simulink model "testemplanner_cs"  (R2023a)
settings: Solver=ode5  StartTime=0.0  StopTime=60  FixedStep=1/1000  RelTol=1e-3
PreLoadFcn:
  | mbxruntime.callbacks.PreLoadFcn(bdroot);
PostLoadFcn:
  | mbxruntime.callbacks.PostLoadFcn(bdroot);
InitFcn:
  | mbxruntime.callbacks.InitFcn(bdroot);
StartFcn:
  | mbxruntime.callbacks.StartFcn(bdroot);
StopFcn:
  | mbxruntime.callbacks.StopFcn(bdroot);
model workspace (MAT data in the model file):
  mbox_table : object (value not decoded)
  model_closed = 0
  sim_status = 0
undefined symbols (not defined in the file): aubr, c_factor, cf, cr, DiscIntNeverNeededParam, global_path_x, global_path_y, KD_PID_distance, KD_PID_speed, KI_PID_distance, KI_PID_speed, KP_PID_distance, KP_PID_speed, la, lb, LQR_K1, LQR_K2, LQR_K3, LQR_K4, m, rack_displacement, right_wheel_ground, tablebr, vubr, vx_break_point
libraries: PreScanSimulinkLibrary x14, Solver_SF x1
(part 8 of 8)

== matlab function testemplanner_cs/Audi_A8_Sedan_1/decision&planning module1/referenceline provider/MATLAB Function ==
  data: path_x input; path_heading output; path_y input; path_kappa output
function [path_heading, path_kappa] = fcn(path_x, path_y)

%原理：heading=atan(dy/dx)
%kappa=dheading/ds
%ds=(dx^2+dy^2)^0.5
%但角度存在多值性问题，例如heading=atan(dy/dx)=heading+pi,在三角函数运算时会出现问题
%可以容忍heading+2pi（三角函数运算不会出现问题），但计算kappa=(dheading+2pi)/ds时要做特殊处理
%很多奇怪问题的根源就是角度的多值性处理不当
%中点欧拉法不能直接用

%dx,dy而不是角度用中点欧拉
dx = diff(path_x);
dy = diff(path_y);

dx_pre = [dx(1);dx];
dx_end = [dx;dx(end)];
dx_final = (dx_pre+dx_end)/2;

dy_pre = [dy(1);dy];
dy_end = [dy;dy(end)];
dy_final = (dy_pre+dy_end)/2;

%.^2是对每一个元素做平方运算，^2是矩阵运算
ds_final = sqrt(dx_final.^2+dy_final.^2);

%atan2为四象限反正切，将角度限定在-pi-pi
path_heading = atan2(dy_final,dx_final);

%对heading做差分，得到dheading，同样采用中点欧拉
dheading = diff(path_heading);
dheading_pre = [dheading(1);dheading];
dheading_after = [dheading;dheading(end)];
dheading_final = (dheading_pre+dheading_after)/2;

%认为dheading为很小量，用sin(dheading)近似代替heading,因为sin(dheading)与sin(dheading+2pi)相等
path_kappa = dheading_final./ds_final;

== matlab function testemplanner_cs/Audi_A8_Sedan_1/decision&planning module1/referenceline provider/MATLAB Function1 ==
  data: host_match_point_index input; referenceline_x_init output; global_path_x input; global_path_y input; referenceline_y_init output
function [referenceline_x_init, referenceline_y_init] = fcn(host_match_point_index, global_path_x, global_path_y)

%提取未经过优化的全局路径
%从自车的匹配点开始，向前取150个点，向后取30个点，总共181个点
%如果后面的点不够30...
%如果前面的点不够150...
%满足条件

start_index = -1;
%后面不足30个点
if host_match_point_index-30 < 1
    start_index = 1;
elseif host_match_point_index+180 > length(global_path_x)
    start_index = length(global_path_x)-180;
else
    start_index = host_match_point_index-29;%可能有问题
end

referenceline_x_init = global_path_x(start_index:start_index+180);
referenceline_y_init = global_path_y(start_index:start_index+180);

== matlab function testemplanner_cs/Audi_A8_Sedan_1/decision&planning module1/referenceline provider/MATLAB Function2 ==
  data: path_x input; path_heading output; path_y input; path_kappa output
function [path_heading, path_kappa] = fcn(path_x, path_y)

%原理：heading=atan(dy/dx)
%kappa=dheading/ds
%ds=(dx^2+dy^2)^0.5
%但角度存在多值性问题，例如heading=atan(dy/dx)=heading+pi,在三角函数运算时会出现问题
%可以容忍heading+2pi（三角函数运算不会出现问题），但计算kappa=(dheading+2pi)/ds时要做特殊处理
%很多奇怪问题的根源就是角度的多值性处理不当
%中点欧拉法不能直接用

%dx,dy而不是角度用中点欧拉
dx = diff(path_x);
dy = diff(path_y);

dx_pre = [dx(1);dx];
dx_end = [dx;dx(end)];
dx_final = (dx_pre+dx_end)/2;

dy_pre = [dy(1);dy];
dy_end = [dy;dy(end)];
dy_final = (dy_pre+dy_end)/2;

%.^2是对每一个元素做平方运算，^2是矩阵运算
ds_final = sqrt(dx_final.^2+dy_final.^2);

%atan2为四象限反正切，将角度限定在-pi-pi
path_heading = atan2(dy_final,dx_final);

%对heading做差分，得到dheading，同样采用中点欧拉
dheading = diff(path_heading);
dheading_pre = [dheading(1);dheading];
dheading_after = [dheading;dheading(end)];
dheading_final = (dheading_pre+dheading_after)/2;

%认为dheading为很小量，用sin(dheading)近似代替heading,因为sin(dheading)与sin(dheading+2pi)相等
path_kappa = dheading_final./ds_final;

== matlab function testemplanner_cs/Audi_A8_Sedan_1/decision&planning module1/referenceline provider/MATLAB Function3 ==
  data: referenceline_x_init input; referenceline_x output; referenceline_y_init input; w_smooth_cost input; w_length_cost input; w_reference_cost input; x_lb input; y_lb input; referenceline_y output; x_ub input; y_ub input
function [referenceline_x, referenceline_y] = fcn(referenceline_x_init, referenceline_y_init, w_smooth_cost, w_length_cost, w_reference_cost, x_lb, y_lb, x_ub, y_ub)

%该模块将xy初始路径通过参考线平滑算法得到参考线
%w_smooth_cost:平滑代价
%w_length_cost:紧凑代价
%w_reference_cost:几何相似度代价
%lb：xy的下界
%ub: xy的上界
%二次规划标准形式：0.5*X'*H*X+f'*X=min
%lb < X <ub
%simulink无法直接调用quadprog,要从外部引入

coder.extrinsic("quadprog");
%一共181个点，对参考线及上下界以及A1A2A3进行初始化
n = 181;
referenceline_x = zeros(n,1);
referenceline_y = zeros(n,1);
lb = zeros(2*n,1);
ub = zeros(2*n,1);

%参考线平滑算法提速
persistent is_first_run
persistent pre_result_x
persistent pre_result_y
persistent pre_referenceline_x_init
persistent pre_referenceline_y_init
if isempty(is_first_run)
    is_first_run = 0;
    
    %对f（参考线初值）及lb，ub进行赋值
    f = zeros(2*n,1);
    for i = 1:n
        %将f的奇数行赋值为参考线x坐标初值
        f(2*i-1) = referenceline_x_init(i);
        %将f的偶数行赋值为参考线y坐标初值
        f(2*i) = referenceline_y_init(i);
        %给上下界lb及ub赋值
        lb(2*i-1) = f(2*i-1)+x_lb;
        lb(2*i) = f(2*i)+y_lb;
        ub(2*i-1) = f(2*i-1)+x_ub;
        ub(2*i) = f(2*i)+y_ub;
    end
    
    %初始化过程矩阵A1并对其赋值,A1为（2n-4）*2n维的矩阵
    %A1 = [1 0 -2 0 1 0
    %        1  0 -2 0 1
    %           1 0 -2 0 1
    %             .................
    A1 = zeros(2*n-4,2*n);
    for j = 1:2*n-5
        A1(j,j) = 1;
        A1(j,j+2) = -2;
        A1(j,j+4) = 1;
        A1(j+1,j+1) = 1;
        A1(j+1,j+3) = -2;
        A1(j+1,j+5) = 1;
    end
    
    %初始化过程矩阵A2并对其进行赋值，A2为（2n-2）*2n维矩阵
    %A2 = [1 0 -1
    %        1 0 -1
    %          1 0 -1
    %            ......
    A2 = zeros(2*n-2,2*n);
    for k = 1:2*n-2
        A2(k,k) = 1;
        A2(k,k+2) = -1;
    end
    
    %初始化过程矩阵A3，A3为2n维单位矩阵
    A3 = eye(2*n);
    
    %将代价函数转化为二次规划的标准形式
    %cost function = X'(w_smooth_cost*A1'*A1+w_length_cost*A2'*A2+w_reference_cost*A3')X+w_reference_cost*h'*X
    %......        = X'HX+f'X
    %......        = 0.5*X'*2H*X+f'X
    H1 = w_smooth_cost*(A1'*A1)+w_length_cost*(A2'*A2)+w_reference_cost*A3';
    H = 2*H1;
    
    %二次规划从参考线初值（f）开始迭代，提高计算效率
    %f = [x1r;y1r;x2r;y2r;...x181r;y181r]
    x0 = f;
    %代入二次规划的标准形式为列向量
    f = -2*w_reference_cost*f;

    X = quadprog(H,f,[],[],[],[],lb,ub,x0);
    %将二次规划的计算结果存储到reference_x及reference_y中
    for m = 1:n
        referenceline_x(m) = X(2*m-1);
        referenceline_y(m) = X(2*m);
    end
    pre_result_x = referenceline_x;
    pre_result_y = referenceline_y;
    pre_referenceline_x_init = referenceline_x_init;
    pre_referenceline_y_init = referenceline_y_init;
else
    if referenceline_x_init(1) == pre_referenceline_x_init(1) && referenceline_y_init(1) == pre_referenceline_y_init(1)
        %初始参考线起点相同则认为平滑后的参考线相同，直接复用上次结果
        referenceline_x = pre_result_x;
        referenceline_y = pre_result_y;
    else        
        %对f（参考线初值）及lb，ub进行赋值
        f = zeros(2*n,1);
        for i = 1:n
            %将f的奇数行赋值为参考线x坐标初值
            f(2*i-1) = referenceline_x_init(i);
            %将f的偶数行赋值为参考线y坐标初值
            f(2*i) = referenceline_y_init(i);
            %给上下界lb及ub赋值
            lb(2*i-1) = f(2*i-1)+x_lb;
            lb(2*i) = f(2*i)+y_lb;
            ub(2*i-1) = f(2*i-1)+x_ub;
            ub(2*i) = f(2*i)+y_ub;
        end
        
        %初始化过程矩阵A1并对其赋值,A1为（2n-4）*2n维的矩阵
        %A1 = [1 0 -2 0 1 0
        %        1  0 -2 0 1
        %           1 0 -2 0 1
        %             .................
        A1 = zeros(2*n-4,2*n);
        for j = 1:2*n-5
            A1(j,j) = 1;
            A1(j,j+2) = -2;
            A1(j,j+4) = 1;
            A1(j+1,j+1) = 1;
            A1(j+1,j+3) = -2;
            A1(j+1,j+5) = 1;
        end
        
        %初始化过程矩阵A2并对其进行赋值，A2为（2n-2）*2n维矩阵
        %A2 = [1 0 -1
        %        1 0 -1
        %          1 0 -1
        %            ......
        A2 = zeros(2*n-2,2*n);
        for k = 1:2*n-2
            A2(k,k) = 1;
            A2(k,k+2) = -1;
        end
        
        %初始化过程矩阵A3，A3为2n维单位矩阵
        A3 = eye(2*n);
        
        %将代价函数转化为二次规划的标准形式
        %cost function = X'(w_smooth_cost*A1'*A1+w_length_cost*A2'*A2+w_reference_cost*A3')X+w_reference_cost*h'*X
        %......        = X'HX+f'X
        %......        = 0.5*X'*2H*X+f'X
        H1 = w_smooth_cost*(A1'*A1)+w_length_cost*(A2'*A2)+w_reference_cost*A3';
        H = 2*H1;
        
        %二次规划从参考线初值（f）开始迭代，提高计算效率
        %f = [x1r;y1r;x2r;y2r;...x181r;y181r]
        x0 = f;
        %代入二次规划的标准形式为列向量
        f = -2*w_reference_cost*f;
    
        X = quadprog(H,f,[],[],[],[],lb,ub,x0);
        %将二次规划的计算结果存储到reference_x及reference_y中
        for m = 1:n
            referenceline_x(m) = X(2*m-1);
            referenceline_y(m) = X(2*m);
        end
        pre_result_x = referenceline_x;
        pre_result_y = referenceline_y;
        pre_referenceline_x_init = referenceline_x_init;
        pre_referenceline_y_init = referenceline_y_init;
    end
end

== matlab function testemplanner_cs/Audi_A8_Sedan_1/decision&planning module1/referenceline provider/MATLAB Function4 ==
  data: path_x input; path_heading output; path_y input; path_kappa output
function [path_heading, path_kappa] = fcn(path_x, path_y)

%原理：heading=atan(dy/dx)
%kappa=dheading/ds
%ds=(dx^2+dy^2)^0.5
%但角度存在多值性问题，例如heading=atan(dy/dx)=heading+pi,在三角函数运算时会出现问题
%可以容忍heading+2pi（三角函数运算不会出现问题），但计算kappa=(dheading+2pi)/ds时要做特殊处理
%很多奇怪问题的根源就是角度的多值性处理不当
%中点欧拉法不能直接用

%dx,dy而不是角度用中点欧拉
dx = diff(path_x);
dy = diff(path_y);

dx_pre = [dx(1);dx];
dx_end = [dx;dx(end)];
dx_final = (dx_pre+dx_end)/2;

dy_pre = [dy(1);dy];
dy_end = [dy;dy(end)];
dy_final = (dy_pre+dy_end)/2;

%.^2是对每一个元素做平方运算，^2是矩阵运算
ds_final = sqrt(dx_final.^2+dy_final.^2);

%atan2为四象限反正切，将角度限定在-pi-pi
path_heading = atan2(dy_final,dx_final);

%对heading做差分，得到dheading，同样采用中点欧拉
dheading = diff(path_heading);
dheading_pre = [dheading(1);dheading];
dheading_after = [dheading;dheading(end)];
dheading_final = (dheading_pre+dheading_after)/2;

%认为dheading为很小量，用sin(dheading)近似代替heading,因为sin(dheading)与sin(dheading+2pi)相等
path_kappa = dheading_final./ds_final;

== matlab function testemplanner_cs/Audi_A8_Sedan_1/decision&planning module1/referenceline provider/match&proj point search1 ==
  data: match_point_index_set output; proj_x_set output; proj_y_set output; proj_heading_set output; proj_kappa_set output; x_set input; y_set input; frenet_x_set input; frenet_y_set input; frenet_heading_set input; frenet_kapppa_set input
function [match_point_index_set, proj_x_set, proj_y_set, proj_heading_set, proj_kappa_set] = fcn(x_set, y_set, frenet_x_set, frenet_y_set, ...
    frenet_heading_set, frenet_kapppa_set)

%待投影点是一个集合（自车，障碍物），每一个点分别遍历寻找匹配点，再寻找投影点
%匹配点集合要保存下来，作为下次遍历开始的起点
%第一次遍历，没有任何提示，从frenet点集第一点开始遍历
%若不是第一次遍历，从上次保存的匹配点开始，注意方向
%待投影点-寻找匹配点-寻找投影点-投影点（x,y,heading,kappa），保存匹配点索引集合

%（待）投影点数量未知，设置缓冲，最多批量处理128个点,信息冗余用NAN（not a number）处理
n = 128;
match_point_index_set = ones(n,1)*nan;
proj_x_set = ones(n,1)*nan;
proj_y_set = ones(n,1)*nan;
proj_heading_set = ones(n,1)*nan;
proj_kappa_set = ones(n,1)*nan;

%两种情况：第一次遍历，非第一次遍历
%声明两个全局变量，第一个用来判断是否初次运行，第二个用来存储上次匹配点集合
persistent is_first_run
persistent pre_match_point_index_set
persistent pre_x_set
persistent pre_y_set
persistent pre_frenet_x_set;
persistent pre_frenet_y_set;
persistent pre_frenet_heading_set;

if isempty(is_first_run)
    is_first_run = 0;
    pre_match_point_index_set = ones(n,1)*nan;
    %遍历每一个点寻找匹配点
    start_search_index = 1;
    for i = 1:length(x_set)
        if isnan(x_set(i))
            break;
        end
        increase_count = 0;
        min_distant = inf;
        for j = start_search_index:length(frenet_x_set)
            distant = (x_set(i)-frenet_x_set(j))^2+(y_set(i)-frenet_y_set(j))^2;
            if distant < min_distant
                min_distant = distant;
                increase_count = 0;
                match_point_index_set(i) = j;
            else
                increase_count = increase_count+1;
            end
            %第一次遍历连续增加50次停止
            if increase_count > 50
                break;
            end
        end
        %通过匹配点计算投影点
        %计算匹配点的位矢及方向向量
        vector_match_point = [frenet_x_set(match_point_index_set(i));frenet_y_set(match_point_index_set(i))];
        vector_match_point_direction = [cos(frenet_heading_set(match_point_index_set(i)));sin(frenet_heading_set(match_point_index_set(i)))];
        vector_d = [x_set(i);y_set(i)]-vector_match_point;
        ds = vector_d'*vector_match_point_direction;
        vector_ds = ds*vector_match_point_direction;
        vector_proj_point = vector_match_point+vector_ds;
        %计算投影点的x,y,heading,kappa
        proj_x_set(i) = vector_proj_point(1);
        proj_y_set(i) = vector_proj_point(2);
        proj_heading_set(i) = frenet_heading_set(match_point_index_set(i))+frenet_kapppa_set(match_point_index_set(i))*ds;
        proj_kappa_set(i) = frenet_kapppa_set(match_point_index_set(i));
    end
    pre_match_point_index_set = match_point_index_set;
    pre_frenet_x_set = frenet_x_set;
    pre_frenet_y_set = frenet_y_set;
    pre_frenet_heading_set = frenet_heading_set;
    pre_x_set = x_set;
    pre_y_set = y_set;
else
    %如果不是第一次遍历
    for i = 1:length(x_set)

        if isnan(x_set(i))
            break;
        end
        %下面这行代码有严重问题，需要投影的不仅是自车，还有障碍物
        %而第一次运行时传感器可能监测不到障碍物，即算法会跳过is first run分支执行else分支
        %此时pre_match_point_index_set中除了自车都是nan，所以需要修复
        start_search_index = pre_match_point_index_set(i);
        increase_count_limit = 5;

        %下面是修复一个bug，pre_match_point_index(i)与x_set(i)不一定是同一个障碍物
        square_dis = (x_set(i)-pre_x_set(i))^2+(y_set(i)-pre_y_set(i))^2;
        if square_dis > 36
            start_search_index = nan;
        end

        if isnan(start_search_index)
            %从第一个点开始遍历，并需要遍历50次防止取到局部极小值
            increase_count_limit = 50;
            start_search_index = 1;
        end

        increase_count = 0;
        min_distant = inf;
        %判断遍历方向
        vector_pre_match_point = [pre_frenet_x_set(start_search_index);pre_frenet_y_set(start_search_index)];
        vector_pre_match_point_direction = [cos(pre_frenet_heading_set(start_search_index));sin(pre_frenet_heading_set(start_search_index))];
        flag = ([x_set(i);y_set(i)]-vector_pre_match_point)'*vector_pre_match_point_direction;
        

        %正向遍历
        if flag > 0.001
            for j = start_search_index:length(frenet_x_set)
                distant = (x_set(i)-frenet_x_set(j))^2+(y_set(i)-frenet_y_set(j))^2;
                if distant < min_distant
                    min_distant = distant;
                    increase_count = 0;
                    match_point_index_set(i) = j;
                else
                    increase_count = increase_count+1;
                end
                %连续增加5次停止
                if increase_count > increase_count_limit
                    break;
                end
            end
            % %通过匹配点计算投影点
            % %计算匹配点的位矢及方向向量
            % vector_match_point = [frenet_x_set(match_point_index_set(i));frenet_y_set(match_point_index_set(i))];
            % vector_match_point_direction = [cos(frenet_heading_set(match_point_index_set(i)));sin(frenet_heading_set(match_point_index_set(i)))];
            % vector_d = [x_set(i);y_set(i)]-vector_match_point;
            % ds = vector_d'*vector_match_point_direction;
            % vector_ds = ds*vector_match_point_direction;
            % vector_proj_point = vector_match_point+vector_ds;
            % %计算投影点的x,y,heading,kappa
            % proj_x_set(i) = vector_proj_point(1);
            % proj_y_set(i) = vector_proj_point(2);
            % proj_heading_set(i) = frenet_heading_set(match_point_index_set(i))+frenet_kapppa_set(match_point_index_set(i))*ds;
            % proj_kappa_set(i) = frenet_kapppa_set(match_point_index_set(i));
        elseif flag < -0.001
            %反向遍历
             for j = start_search_index:-1:1
                distant = (x_set(i)-frenet_x_set(j))^2+(y_set(i)-frenet_y_set(j))^2;
                if distant < min_distant
                    min_distant = distant;
                    increase_count = 0;
                    match_point_index_set(i) = j;
                else
                    increase_count = increase_count+1;
                end
                %连续增加5次停止
                if increase_count > increase_count_limit
                    break;
                end
            end
        else
            match_point_index_set(i) = start_search_index;
        end

        %通过匹配点计算投影点
        %计算匹配点的位矢及方向向量
        vector_match_point = [frenet_x_set(match_point_index_set(i));frenet_y_set(match_point_index_set(i))];
        vector_match_point_direction = [cos(frenet_heading_set(match_point_index_set(i)));sin(frenet_heading_set(match_point_index_set(i)))];
        vector_d = [x_set(i);y_set(i)]-vector_match_point;
        ds = vector_d'*vector_match_point_direction;
        vector_ds = ds*vector_match_point_direction;
        vector_proj_point = vector_match_point+vector_ds;
        %计算投影点的x,y,heading,kappa
        proj_x_set(i) = vector_proj_point(1);
        proj_y_set(i) = vector_proj_point(2);
        proj_heading_set(i) = frenet_heading_set(match_point_index_set(i))+frenet_kapppa_set(match_point_index_set(i))*ds;
        proj_kappa_set(i) = frenet_kapppa_set(match_point_index_set(i));

    end
    pre_match_point_index_set = match_point_index_set;
    pre_frenet_x_set = frenet_x_set;
    pre_frenet_y_set = frenet_y_set;
    pre_frenet_heading_set = frenet_heading_set;
    pre_x_set = x_set;
    pre_y_set = y_set;
end

== matlab function testemplanner_cs/Audi_A8_Sedan_1/decision&planning module1/referenceline provider/match&proj point search2 ==
  data: match_point_index_set output; proj_x_set output; proj_y_set output; proj_heading_set output; proj_kappa_set output; x_set input; y_set input; frenet_x_set input; frenet_y_set input; frenet_heading_set input; frenet_kapppa_set input
function [match_point_index_set, proj_x_set, proj_y_set, proj_heading_set, proj_kappa_set] = fcn(x_set, y_set, frenet_x_set, frenet_y_set, ...
    frenet_heading_set, frenet_kapppa_set)

%待投影点是一个集合（自车，障碍物），每一个点分别遍历寻找匹配点，再寻找投影点
%匹配点集合要保存下来，作为下次遍历开始的起点
%第一次遍历，没有任何提示，从frenet点集第一点开始遍历
%若不是第一次遍历，从上次保存的匹配点开始，注意方向
%待投影点-寻找匹配点-寻找投影点-投影点（x,y,heading,kappa），保存匹配点索引集合

%（待）投影点数量未知，设置缓冲，最多批量处理128个点,信息冗余用NAN（not a number）处理
n = 128;
match_point_index_set = ones(n,1)*nan;
proj_x_set = ones(n,1)*nan;
proj_y_set = ones(n,1)*nan;
proj_heading_set = ones(n,1)*nan;
proj_kappa_set = ones(n,1)*nan;

%两种情况：第一次遍历，非第一次遍历
%声明两个全局变量，第一个用来判断是否初次运行，第二个用来存储上次匹配点集合
persistent is_first_run
persistent pre_match_point_index_set
persistent pre_x_set
persistent pre_y_set
persistent pre_frenet_x_set;
persistent pre_frenet_y_set;
persistent pre_frenet_heading_set;

if isempty(is_first_run)
    is_first_run = 0;
    pre_match_point_index_set = ones(n,1)*nan;
    %遍历每一个点寻找匹配点
    start_search_index = 1;
    for i = 1:length(x_set)
        if isnan(x_set(i))
            break;
        end
        increase_count = 0;
        min_distant = inf;
        for j = start_search_index:length(frenet_x_set)
            distant = (x_set(i)-frenet_x_set(j))^2+(y_set(i)-frenet_y_set(j))^2;
            if distant < min_distant
                min_distant = distant;
                increase_count = 0;
                match_point_index_set(i) = j;
            else
                increase_count = increase_count+1;
            end
            %第一次遍历连续增加50次停止
            if increase_count > 50
                break;
            end
        end
        %通过匹配点计算投影点
        %计算匹配点的位矢及方向向量
        vector_match_point = [frenet_x_set(match_point_index_set(i));frenet_y_set(match_point_index_set(i))];
        vector_match_point_direction = [cos(frenet_heading_set(match_point_index_set(i)));sin(frenet_heading_set(match_point_index_set(i)))];
        vector_d = [x_set(i);y_set(i)]-vector_match_point;
        ds = vector_d'*vector_match_point_direction;
        vector_ds = ds*vector_match_point_direction;
        vector_proj_point = vector_match_point+vector_ds;
        %计算投影点的x,y,heading,kappa
        proj_x_set(i) = vector_proj_point(1);
        proj_y_set(i) = vector_proj_point(2);
        proj_heading_set(i) = frenet_heading_set(match_point_index_set(i))+frenet_kapppa_set(match_point_index_set(i))*ds;
        proj_kappa_set(i) = frenet_kapppa_set(match_point_index_set(i));
    end
    pre_match_point_index_set = match_point_index_set;
    pre_frenet_x_set = frenet_x_set;
    pre_frenet_y_set = frenet_y_set;
    pre_frenet_heading_set = frenet_heading_set;
    pre_x_set = x_set;
    pre_y_set = y_set;
else
    %如果不是第一次遍历
    for i = 1:length(x_set)

        if isnan(x_set(i))
            break;
        end
        %下面这行代码有严重问题，需要投影的不仅是自车，还有障碍物
        %而第一次运行时传感器可能监测不到障碍物，即算法会跳过is first run分支执行else分支
        %此时pre_match_point_index_set中除了自车都是nan，所以需要修复
        start_search_index = pre_match_point_index_set(i);
        increase_count_limit = 5;

        %下面是修复一个bug，pre_match_point_index(i)与x_set(i)不一定是同一个障碍物
        square_dis = (x_set(i)-pre_x_set(i))^2+(y_set(i)-pre_y_set(i))^2;
        if square_dis > 36
            start_search_index = nan;
        end

        if isnan(start_search_index)
            %从第一个点开始遍历，并需要遍历50次防止取到局部极小值
            increase_count_limit = 50;
            start_search_index = 1;
        end

        increase_count = 0;
        min_distant = inf;
        %判断遍历方向
        vector_pre_match_point = [pre_frenet_x_set(start_search_index);pre_frenet_y_set(start_search_index)];
        vector_pre_match_point_direction = [cos(pre_frenet_heading_set(start_search_index));sin(pre_frenet_heading_set(start_search_index))];
        flag = ([x_set(i);y_set(i)]-vector_pre_match_point)'*vector_pre_match_point_direction;
        

        %正向遍历
        if flag > 0.001
            for j = start_search_index:length(frenet_x_set)
                distant = (x_set(i)-frenet_x_set(j))^2+(y_set(i)-frenet_y_set(j))^2;
                if distant < min_distant
                    min_distant = distant;
                    increase_count = 0;
                    match_point_index_set(i) = j;
                else
                    increase_count = increase_count+1;
                end
                %连续增加5次停止
                if increase_count > increase_count_limit
                    break;
                end
            end
            % %通过匹配点计算投影点
            % %计算匹配点的位矢及方向向量
            % vector_match_point = [frenet_x_set(match_point_index_set(i));frenet_y_set(match_point_index_set(i))];
            % vector_match_point_direction = [cos(frenet_heading_set(match_point_index_set(i)));sin(frenet_heading_set(match_point_index_set(i)))];
            % vector_d = [x_set(i);y_set(i)]-vector_match_point;
            % ds = vector_d'*vector_match_point_direction;
            % vector_ds = ds*vector_match_point_direction;
            % vector_proj_point = vector_match_point+vector_ds;
            % %计算投影点的x,y,heading,kappa
            % proj_x_set(i) = vector_proj_point(1);
            % proj_y_set(i) = vector_proj_point(2);
            % proj_heading_set(i) = frenet_heading_set(match_point_index_set(i))+frenet_kapppa_set(match_point_index_set(i))*ds;
            % proj_kappa_set(i) = frenet_kapppa_set(match_point_index_set(i));
        elseif flag < -0.001
            %反向遍历
             for j = start_search_index:-1:1
                distant = (x_set(i)-frenet_x_set(j))^2+(y_set(i)-frenet_y_set(j))^2;
                if distant < min_distant
                    min_distant = distant;
                    increase_count = 0;
                    match_point_index_set(i) = j;
                else
                    increase_count = increase_count+1;
                end
                %连续增加5次停止
                if increase_count > increase_count_limit
                    break;
                end
            end
        else
            match_point_index_set(i) = start_search_index;
        end

        %通过匹配点计算投影点
        %计算匹配点的位矢及方向向量
        vector_match_point = [frenet_x_set(match_point_index_set(i));frenet_y_set(match_point_index_set(i))];
        vector_match_point_direction = [cos(frenet_heading_set(match_point_index_set(i)));sin(frenet_heading_set(match_point_index_set(i)))];
        vector_d = [x_set(i);y_set(i)]-vector_match_point;
        ds = vector_d'*vector_match_point_direction;
        vector_ds = ds*vector_match_point_direction;
        vector_proj_point = vector_match_point+vector_ds;
        %计算投影点的x,y,heading,kappa
        proj_x_set(i) = vector_proj_point(1);
        proj_y_set(i) = vector_proj_point(2);
        proj_heading_set(i) = frenet_heading_set(match_point_index_set(i))+frenet_kapppa_set(match_point_index_set(i))*ds;
        proj_kappa_set(i) = frenet_kapppa_set(match_point_index_set(i));

    end
    pre_match_point_index_set = match_point_index_set;
    pre_frenet_x_set = frenet_x_set;
    pre_frenet_y_set = frenet_y_set;
    pre_frenet_heading_set = frenet_heading_set;
    pre_x_set = x_set;
    pre_y_set = y_set;
end

== matlab function testemplanner_cs/Audi_A8_Sedan_1/decision&planning module1/referenceline provider/match&proj point search3 ==
  data: match_point_index_set output; proj_x_set output; proj_y_set output; proj_heading_set output; proj_kappa_set output; x_set input; y_set input; frenet_x_set input; frenet_y_set input; frenet_heading_set input; frenet_kapppa_set input
function [match_point_index_set, proj_x_set, proj_y_set, proj_heading_set, proj_kappa_set] = fcn(x_set, y_set, frenet_x_set, frenet_y_set, ...
    frenet_heading_set, frenet_kapppa_set)

%待投影点是一个集合（自车，障碍物），每一个点分别遍历寻找匹配点，再寻找投影点
%匹配点集合要保存下来，作为下次遍历开始的起点
%第一次遍历，没有任何提示，从frenet点集第一点开始遍历
%若不是第一次遍历，从上次保存的匹配点开始，注意方向
%待投影点-寻找匹配点-寻找投影点-投影点（x,y,heading,kappa），保存匹配点索引集合

%（待）投影点数量未知，设置缓冲，最多批量处理128个点,信息冗余用NAN（not a number）处理
n = 128;
match_point_index_set = ones(n,1)*nan;
proj_x_set = ones(n,1)*nan;
proj_y_set = ones(n,1)*nan;
proj_heading_set = ones(n,1)*nan;
proj_kappa_set = ones(n,1)*nan;

%两种情况：第一次遍历，非第一次遍历
%声明两个全局变量，第一个用来判断是否初次运行，第二个用来存储上次匹配点集合
persistent is_first_run
persistent pre_match_point_index_set

if isempty(is_first_run)
    is_first_run = 0;
    pre_match_point_index_set = ones(n,1)*nan;
    %遍历每一个点寻找匹配点
    start_search_index = 1;
    for i = 1:length(x_set)
        if isnan(x_set(i))
            break;
        end
        increase_count = 0;
        min_distant = inf;
        for j = start_search_index:length(frenet_x_set)
            distant = (x_set(i)-frenet_x_set(j))^2+(y_set(i)-frenet_y_set(j))^2;
            if distant < min_distant
                min_distant = distant;
                increase_count = 0;
                match_point_index_set(i) = j;
            else
                increase_count = increase_count+1;
            end
            %第一次遍历连续增加50次停止
            if increase_count > 50
                break;
            end
        end
        %通过匹配点计算投影点
        %计算匹配点的位矢及方向向量
        vector_match_point = [frenet_x_set(match_point_index_set(i));frenet_y_set(match_point_index_set(i))];
        vector_match_point_direction = [cos(frenet_heading_set(match_point_index_set(i)));sin(frenet_heading_set(match_point_index_set(i)))];
        vector_d = [x_set(i);y_set(i)]-vector_match_point;
        ds = vector_d'*vector_match_point_direction;
        vector_ds = ds*vector_match_point_direction;
        vector_proj_point = vector_match_point+vector_ds;
        %计算投影点的x,y,heading,kappa
        proj_x_set(i) = vector_proj_point(1);
        proj_y_set(i) = vector_proj_point(2);
        proj_heading_set(i) = frenet_heading_set(match_point_index_set(i))+frenet_kapppa_set(match_point_index_set(i))*ds;
        proj_kappa_set(i) = frenet_kapppa_set(match_point_index_set(i));
    end
    pre_match_point_index_set = match_point_index_set;
else
    %如果不是第一次遍历
    for i = 1:length(x_set)

        if isnan(x_set(i))
            break;
        end
        %下面这行代码有严重问题，需要投影的不仅是自车，还有障碍物
        %而第一次运行时传感器可能监测不到障碍物，即算法会跳过is first run分支执行else分支
        %此时pre_match_point_index_set中除了自车都是nan，所以需要修复
        start_search_index = pre_match_point_index_set(i);
        increase_count_limit = 5;

        if isnan(start_search_index)
            %从第一个点开始遍历，并需要遍历50次防止取到局部极小值
            increase_count_limit = 50;
            start_search_index = 1;
        end

        increase_count = 0;
        min_distant = inf;
        %判断遍历方向
        vector_pre_match_point = [frenet_x_set(start_search_index);frenet_y_set(start_search_index)];
        vector_pre_match_point_direction = [cos(frenet_heading_set(start_search_index));sin(frenet_heading_set(start_search_index))];
        flag = ([x_set(i);y_set(i)]-vector_pre_match_point)'*vector_pre_match_point_direction;
        

        %正向遍历
        if flag > 0.001
            for j = start_search_index:length(frenet_x_set)
                distant = (x_set(i)-frenet_x_set(j))^2+(y_set(i)-frenet_y_set(j))^2;
                if distant < min_distant
                    min_distant = distant;
                    increase_count = 0;
                    match_point_index_set(i) = j;
                else
                    increase_count = increase_count+1;
                end
                %连续增加5次停止
                if increase_count > increase_count_limit
                    break;
                end
            end
            % %通过匹配点计算投影点
            % %计算匹配点的位矢及方向向量
            % vector_match_point = [frenet_x_set(match_point_index_set(i));frenet_y_set(match_point_index_set(i))];
            % vector_match_point_direction = [cos(frenet_heading_set(match_point_index_set(i)));sin(frenet_heading_set(match_point_index_set(i)))];
            % vector_d = [x_set(i);y_set(i)]-vector_match_point;
            % ds = vector_d'*vector_match_point_direction;
            % vector_ds = ds*vector_match_point_direction;
            % vector_proj_point = vector_match_point+vector_ds;
            % %计算投影点的x,y,heading,kappa
            % proj_x_set(i) = vector_proj_point(1);
            % proj_y_set(i) = vector_proj_point(2);
            % proj_heading_set(i) = frenet_heading_set(match_point_index_set(i))+frenet_kapppa_set(match_point_index_set(i))*ds;
            % proj_kappa_set(i) = frenet_kapppa_set(match_point_index_set(i));
        elseif flag < -0.001
            %反向遍历
             for j = start_search_index:-1:1
                distant = (x_set(i)-frenet_x_set(j))^2+(y_set(i)-frenet_y_set(j))^2;
                if distant < min_distant
                    min_distant = distant;
                    increase_count = 0;
                    match_point_index_set(i) = j;
                else
                    increase_count = increase_count+1;
                end
                %连续增加5次停止
                if increase_count > increase_count_limit
                    break;
                end
            end
        else
            match_point_index_set(i) = start_search_index;
        end

        %通过匹配点计算投影点
        %计算匹配点的位矢及方向向量
        vector_match_point = [frenet_x_set(match_point_index_set(i));frenet_y_set(match_point_index_set(i))];
        vector_match_point_direction = [cos(frenet_heading_set(match_point_index_set(i)));sin(frenet_heading_set(match_point_index_set(i)))];
        vector_d = [x_set(i);y_set(i)]-vector_match_point;
        ds = vector_d'*vector_match_point_direction;
        vector_ds = ds*vector_match_point_direction;
        vector_proj_point = vector_match_point+vector_ds;
        %计算投影点的x,y,heading,kappa
        proj_x_set(i) = vector_proj_point(1);
        proj_y_set(i) = vector_proj_point(2);
        proj_heading_set(i) = frenet_heading_set(match_point_index_set(i))+frenet_kapppa_set(match_point_index_set(i))*ds;
        proj_kappa_set(i) = frenet_kapppa_set(match_point_index_set(i));

    end
    pre_match_point_index_set = match_point_index_set;
end

== matlab function testemplanner_cs/Audi_A8_Sedan_1/Perception Provider/MATLAB Function ==
  data: obs_x_set_gcs output; obs_y_set_gcs output; obs_velocity_set_gcs output; obs_heading_set_gcs output; host_x input; host_y input; host_xy_heading input; obs_range input; obs_theta input; obs_velocity input; obs_heading input
function [obs_x_set_gcs, obs_y_set_gcs, obs_velocity_set_gcs, obs_heading_set_gcs] = fcn(host_x, host_y, host_xy_heading, ...
    obs_range, obs_theta, obs_velocity, obs_heading)

%gcs为global coordinate system,即笛卡尔坐标系
%函数输入：
% host x定位在笛卡尔坐标系下的x坐标，host_y定位在笛卡尔坐标系下的y坐标，host_xy_heading:航向角
%obs_range:传感器到障碍物几何中心的距离，obs_theta:极坐标下坐标轴到range方向的角度
%obs_velocity:障碍物的绝对速度
%obs_heading:障碍物速度方向到坐标轴（N轴）的航向角
%输出：
% obs_xset_gcs:障碍物在笛卡尔坐标系下x坐标的集合
% obs_yset_gcs:....................y坐标.....
% obs_velocityset_gcs:.............速度......
% obs_headingset_gcs:..............速度的航向角的集合
% 注意坐标轴变换及单位变换，prescan输出的角度单位是rad

%传感器能识别最多32个障碍物，但事先不知道有多少障碍物，要做缓冲
obs_x_set_gcs = ones(32,1)*nan;
obs_y_set_gcs = ones(32,1)*nan;
obs_velocity_set_gcs = ones(32,1)*nan;
obs_heading_set_gcs = ones(32,1)*nan;

%在prescan的极坐标下顺时针为正，而我们认为逆时针为正
transfer_theta = -obs_theta.*pi/180;
transfer_velocity = obs_velocity;
transfer_heading = (90*ones(32,1)-obs_heading).*pi/180;
transfer_range_x = obs_range.*cos(transfer_theta+host_xy_heading);
transfer_range_y = obs_range.*sin(transfer_theta+host_xy_heading);

%计算障碍物在笛卡尔坐标系下的x,y,heading,velocity
%transfer_range是传感器到障碍物几何中心的距离，还需要考虑传感器到车辆中心的距离
%经过测算，传感器到车辆中心的距离大概是2.173
for i = 1:32
    %判断第i个障碍物是否存在
    if obs_range(i) ~= 0
        obs_x_set_gcs(i) = transfer_range_x(i)+host_x+2.173*cos(host_xy_heading);
        obs_y_set_gcs(i) = transfer_range_y(i)+host_y+2.173*sin(host_xy_heading);
        obs_velocity_set_gcs(i) = transfer_velocity(i);
        obs_heading_set_gcs(i) = transfer_heading(i);
    end
end

== matlab function testemplanner_cs/Audi_A8_Sedan_1/control module/control main/lateral control LQR/err_kappa_calculate_module ==
  data: x input; y input; phi input; vx input; vy input; phi_dot input; xr input; yr input; thetar input; kappar input; err output; es output; s_dot output
function [err,es,s_dot] = fcn(x,y,phi,vx,vy,phi_dot,xr,yr,thetar,kappar)
    
    tor=[cos(thetar);sin(thetar)];
    nor=[-sin(thetar);cos(thetar)];
    d_err=[x-xr;y-yr];
    ed=nor'*d_err;
    es=tor'*d_err;
    %projection_point_thetar=thetar(dmin);%apollo
    projection_point_thetar=thetar+kappar*es;
    ed_dot=vy*cos(phi-projection_point_thetar)+vx*sin(phi-projection_point_thetar);
    %%%%%%%%%
    ephi=sin(phi-projection_point_thetar);
    %%%%%%%%%
    ss_dot=vx*cos(phi-projection_point_thetar)-vy*sin(phi-projection_point_thetar);
    s_dot=ss_dot/(1-kappar*ed);
    ephi_dot=phi_dot-kappar*s_dot;
    err=[ed;ed_dot;ephi;ephi_dot];
    
    
    
    
    
    
    
    
    
    
    
    


end
